simulink library "intertravamento"  (R2015a)
settings: Solver=ode45  SolverMode=SingleTasking  StartTime=0.0  StopTime=10.0  RelTol=1e-3
PostLoadFcn:
  | setsysloc_simulink(bdroot)
undefined symbols (not defined in the file or in its folder): docblock, getdatatypespecs, NumBits1, NumBits2, sfunxy, sigbuilder_block, slcm, SlDemoSign, Slope1, Slope2
libraries: simulink x46, sl_helperblocks x2, eml_lib x1
(part 2 of 6)

== system intertravamento/Continuous ==
  note: Integrators
  note: Delays
  note: Transfer Functions
  note: PID Controllers
  note: Derivative
  Derivative : Derivative
  Integrator : Integrator
  Integrator Limited : Integrator  LimitOutput=on  UpperSaturationLimit=1  LowerSaturationLimit=0
  "Integrator, Second-Order" : SecondOrderIntegrator
  "Integrator, Second-Order Limited" : SecondOrderIntegrator  LimitX=on  UpperLimitX=1  LowerLimitX=0  LimitDXDT=on
  PID Controller : Subsystem  DialogController=pidpack.PIDConfig.pidDDGCreate  mask(PID 1dof){Controller=PID, TimeDomain=Continuous-time, SampleTime=-1, IntegratorMethod=Forward Euler, FilterMethod=Forward Euler, Form=Parallel, UseFilter=on, ControllerParametersSource=internal, P=1, I=1, D=0, N=100, InitialConditionSource=internal, InitialConditionForIntegrator=0, InitialConditionForFilter=0, ExternalReset=none, IgnoreLimit=off, ZeroCross=on, LimitOutput=off, UpperSaturationLimit=inf, LowerSaturationLimit=-inf, LinearizeAsGain=on, AntiWindupMode=none, Kb=1, TrackingMode=off, Kt=1, RndMeth=Floor, SaturateOnIntegerOverflow=off, LockScale=off, PParamMin=[], PParamMax=[], PParamDataTypeStr=Inherit: Inherit via internal rule, IParamMin=[], IParamMax=[], IParamDataTypeStr=Inherit: Inherit via internal rule, DParamMin=[], DParamMax=[], DParamDataTypeStr=Inherit: Inherit via internal rule, NParamMin=[], NParamMax=[], NParamDataTypeStr=Inherit: Inherit via internal rule, KbParamMin=[], KbParamMax=[], KbParamDataTypeStr=Inherit: Inherit via internal rule, KtParamMin=[], KtParamMax=[], KtParamDataTypeStr=Inherit: Inherit via internal rule, POutMin=[], POutMax=[], POutDataTypeStr=Inherit: Inherit via internal rule, PGainOutDataTypeStr=Inherit: Inherit via internal rule, PProdOutDataTypeStr=Inherit: Inherit via internal rule, IOutMin=[], IOutMax=[], IOutDataTypeStr=Inherit: Inherit via internal rule, IGainOutDataTypeStr=Inherit: Inherit via internal rule, IProdOutDataTypeStr=Inherit: Inherit via internal rule, DOutMin=[], DOutMax=[], DOutDataTypeStr=Inherit: Inherit via internal rule, DGainOutDataTypeStr=Inherit: Inherit via internal rule, DProdOutDataTypeStr=Inherit: Inherit via internal rule, NOutMin=[], NOutMax=[], NOutDataTypeStr=Inherit: Inherit via internal rule, NGainOutDataTypeStr=Inherit: Inherit via internal rule, NProdOutDataTypeStr=Inherit: Inherit via internal rule, KbOutMin=[], KbOutMax=[], KbOutDataTypeStr=Inherit: Inherit via internal rule, KtOutMin=[], KtOutMax=[], KtOutDataTypeStr=Inherit: Inherit via internal rule, IntegratorOutMin=[], IntegratorOutMax=[], IntegratorOutDataTypeStr=Inherit: Inherit via internal rule, FilterOutMin=[], FilterOutMax=[], FilterOutDataTypeStr=Inherit: Inherit via internal rule, SumOutMin=[], SumOutMax=[], SumOutDataTypeStr=Inherit: Inherit via internal rule, SumI1OutMin=[], SumI1OutMax=[], SumI1OutDataTypeStr=Inherit: Inherit via internal rule, SumI2OutMin=[], SumI2OutMax=[], SumI2OutDataTypeStr=Inherit: Inherit via internal rule, SumI3OutMin=[], SumI3OutMax=[], SumI3OutDataTypeStr=Inherit: Inherit via internal rule, SumDOutMin=[], SumDOutMax=[], SumDOutDataTypeStr=Inherit: Inherit via internal rule, SumAccumDataTypeStr=Inherit: Inherit via internal rule, SumI1AccumDataTypeStr=Inherit: Inherit via internal rule, SumI2AccumDataTypeStr=Inherit: Inherit via internal rule, SumI3AccumDataTypeStr=Inherit: Inherit via internal rule, SumDAccumDataTypeStr=Inherit: Inherit via internal rule, SaturationOutMin=[], SaturationOutMax=[], SaturationOutDataTypeStr=Inherit: Same as input, IntegratorContinuousStateAttributes='', IntegratorStateIdentifier=, IntegratorStateMustResolveToSignalObject=off, IntegratorRTWStateStorageClass=Auto, IntegratorRTWStateStorageTypeQualifier=, FilterContinuousStateAttributes='', FilterStateIdentifier=, FilterStateMustResolveToSignalObject=off, FilterRTWStateStorageClass=Auto, FilterRTWStateStorageTypeQualifier=, DifferentiatorICPrevScaledInput=0, DifferentiatorOutMin=[], DifferentiatorOutMax=[], DifferentiatorOutDataTypeStr=Inherit: Inherit via internal rule}
      mask prompts: Controller "Simulink:masks:Controller_MP"; TimeDomain "Simulink:masks:TimeDomain_MP"; SampleTime "Simulink:masks:SampleTime1ForInherited_MP"; IntegratorMethod "Simulink:masks:IntegratorMethod_MP"; FilterMethod "Simulink:masks:FilterMethod_MP"; Form "Simulink:masks:Form_MP"; UseFilter "Simulink:masks:UseFilter_MP"; ControllerParametersSource "Simulink:masks:Source_MP"; P "Simulink:masks:ProportionalP_MP"; I "Simulink:masks:IntegralI_MP"; D "Simulink:masks:DerivativeD_MP"; N "Simulink:masks:FilterCoefficientN_MP"; InitialConditionSource "Simulink:masks:Source_MP"; InitialConditionForIntegrator "Simulink:masks:Integrator_MP"; InitialConditionForFilter "Simulink:masks:Filter_MP"; ExternalReset "Simulink:masks:ExternalReset_MP"; IgnoreLimit "Simulink:masks:IgnoreResetWhenLinearizing_MP"; ZeroCross "Simulink:masks:EnableZerocrossingDetection_MP"; LimitOutput "Simulink:masks:LimitOutput_MP"; UpperSaturationLimit "Simulink:masks:UpperSaturationLimit_MP"; LowerSaturationLimit "Simulink:masks:LowerSaturationLimit_MP"; LinearizeAsGain "Simulink:masks:IgnoreSaturationWhenLinearizing_MP"; AntiWindupMode "Simulink:masks:AntiwindupMethod_MP"; Kb "Simulink:masks:BackcalculationCoefficientKb_MP"; TrackingMode "Simulink:masks:EnableTrackingMode_MP"; Kt "Simulink:masks:TrackingCoefficientKt_MP"; RndMeth "Simulink:masks:IntegerRoundingMode_MP"; SaturateOnIntegerOverflow "Simulink:masks:SaturateOnIntegerOverflow_MP"; LockScale "Simulink:masks:LockDataTypeAgainstFxpTools_MP"; PParamMin "Simulink:masks:PParameterMinimum_MP"; PParamMax "Simulink:masks:PParameterMaximum_MP"; PParamDataTypeStr "Simulink:masks:PParameter_MP"; IParamMin "Simulink:masks:IParameterMinimum_MP"; IParamMax "Simulink:masks:IParameterMaximum_MP"; IParamDataTypeStr "Simulink:masks:IParameter_MP"; DParamMin "Simulink:masks:DParameterMinimum_MP"; DParamMax "Simulink:masks:DParameterMaximum_MP"; DParamDataTypeStr "Simulink:masks:DParameter_MP"; NParamMin "Simulink:masks:NParameterMinimum_MP"; NParamMax "Simulink:masks:NParameterMaximum_MP"; NParamDataTypeStr "Simulink:masks:NParameter_MP"; KbParamMin "Simulink:masks:KbParameterMinimum_MP"; KbParamMax "Simulink:masks:KbParameterMaximum_MP"; KbParamDataTypeStr "Simulink:masks:KbParameter_MP"; KtParamMin "Simulink:masks:KtParameterMinimum_MP"; KtParamMax "Simulink:masks:KtParameterMaximum_MP"; KtParamDataTypeStr "Simulink:masks:KtParameter_MP"; POutMin "Simulink:masks:PProductOutputMinimum_MP"; POutMax "Simulink:masks:PProductOutputMaximum_MP"; POutDataTypeStr "Simulink:masks:PProductOutput_MP"; PGainOutDataTypeStr "Simulink:masks:PProductOutput_MP"; PProdOutDataTypeStr "Simulink:masks:PProductOutput_MP"; IOutMin "Simulink:masks:IProductOutputMinimum_MP"; IOutMax "Simulink:masks:IProductOutputMaximum_MP"; IOutDataTypeStr "Simulink:masks:IProductOutput_MP"; IGainOutDataTypeStr "Simulink:masks:IProductOutput_MP"; IProdOutDataTypeStr "Simulink:masks:IProductOutput_MP"; DOutMin "Simulink:masks:DProductOutputMinimum_MP"; DOutMax "Simulink:masks:DProductOutputMaximum_MP"; DOutDataTypeStr "Simulink:masks:DProductOutput_MP"; DGainOutDataTypeStr "Simulink:masks:DProductOutput_MP"; DProdOutDataTypeStr "Simulink:masks:DProductOutput_MP"; NOutMin "Simulink:masks:NProductOutputMinimum_MP"; NOutMax "Simulink:masks:NProductOutputMaximum_MP"; NOutDataTypeStr "Simulink:masks:NProductOutput_MP"; NGainOutDataTypeStr "Simulink:masks:NProductOutput_MP"; NProdOutDataTypeStr "Simulink:masks:NProductOutput_MP"; KbOutMin "Simulink:masks:KbProductOutputMinimum_MP"; KbOutMax "Simulink:masks:KbProductOutputMaximum_MP"; KbOutDataTypeStr "Simulink:masks:KbProductOutput_MP"; KtOutMin "Simulink:masks:KtProductOutputMinimum_MP"; KtOutMax "Simulink:masks:KtProductOutputMaximum_MP"; KtOutDataTypeStr "Simulink:masks:KtProductOutput_MP"; IntegratorOutMin "Simulink:masks:IntegratorOutputMinimum_MP"; IntegratorOutMax "Simulink:masks:IntegratorOutputMaximum_MP"; IntegratorOutDataTypeStr "Simulink:masks:IntegratorOutput_MP"; FilterOutMin "Simulink:masks:FilterOutputMinimum_MP"; FilterOutMax "Simulink:masks:FilterOutputMaximum_MP"; FilterOutDataTypeStr "Simulink:masks:FilterOutput_MP"; SumOutMin "Simulink:masks:SumOutputMinimum_MP"; SumOutMax "Simulink:masks:SumOutputMaximum_MP"; SumOutDataTypeStr "Simulink:masks:SumOutput_MP"; SumI1OutMin "Simulink:masks:SumI1OutputMinimum_MP"; SumI1OutMax "Simulink:masks:SumI1OutputMaximum_MP"; SumI1OutDataTypeStr "Simulink:masks:SumI1Output_MP"; SumI2OutMin "Simulink:masks:SumI2OutputMinimum_MP"; SumI2OutMax "Simulink:masks:SumI2OutputMaximum_MP"; SumI2OutDataTypeStr "Simulink:masks:SumI2Output_MP"; SumI3OutMin "Simulink:masks:SumI3OutputMinimum_MP"; SumI3OutMax "Simulink:masks:SumI3OutputMaximum_MP"; SumI3OutDataTypeStr "Simulink:masks:SumI3Output_MP"; SumDOutMin "Simulink:masks:SumDOutputMinimum_MP"; SumDOutMax "Simulink:masks:SumDOutputMaximum_MP"; SumDOutDataTypeStr "Simulink:masks:SumDOutput_MP"; SumAccumDataTypeStr "Simulink:masks:AccumulatorOfSum_MP"; SumI1AccumDataTypeStr "Simulink:masks:AccumulatorOfSumI1_MP"; SumI2AccumDataTypeStr "Simulink:masks:AccumulatorOfSumI2_MP"; SumI3AccumDataTypeStr "Simulink:masks:AccumulatorOfSumI3_MP"; SumDAccumDataTypeStr "Simulink:masks:AccumulatorOfSumD_MP"; SaturationOutMin "Simulink:masks:SaturationOutputMinimum_MP"; SaturationOutMax "Simulink:masks:SaturationOutputMaximum_MP"; SaturationOutDataTypeStr "Simulink:masks:SaturationOutput_MP"; IntegratorContinuousStateAttributes "Simulink:masks:StateNameegposition_MP"; IntegratorStateIdentifier "Simulink:masks:StateName_MP"; IntegratorStateMustResolveToSignalObject "Simulink:masks:StateNameMustResolveToSimulinkSignalObject_MP"; IntegratorRTWStateStorageClass "Simulink:masks:CodeGenerationStorageClass_MP"; IntegratorRTWStateStorageTypeQualifier "Simulink:masks:CodeGenerationStorageTypeQualifier_MP"; FilterContinuousStateAttributes "Simulink:masks:StateNameegposition_MP"; FilterStateIdentifier "Simulink:masks:StateName_MP"; FilterStateMustResolveToSignalObject "Simulink:masks:StateNameMustResolveToSimulinkSignalObject_MP"; FilterRTWStateStorageClass "Simulink:masks:CodeGenerationStorageClass_MP"; FilterRTWStateStorageTypeQualifier "Simulink:masks:CodeGenerationStorageTypeQualifier_MP"; DifferentiatorICPrevScaledInput "Simulink:masks:Differentiator_MP"; DifferentiatorOutMin "Simulink:masks:DifferentiatorOutputMinimum_MP"; DifferentiatorOutMax "Simulink:masks:DifferentiatorOutputMaximum_MP"; DifferentiatorOutDataTypeStr "Simulink:masks:DifferentiatorOutput_MP"
      mask help: Simulink:masks:PID1dof_MD
      mask init:
      | pidpack.PIDConfig.configPID(gcbh);
      settings: DeleteFcn=pidpack.PIDConfig.closeTuner(gcbh)  ModelCloseFcn=pidpack.PIDConfig.closeTuner(gcbh)  NameChangeFcn=pidpack.PIDConfig.updateTunerName(gcbh)
      mask TypeOptions Controller: Simulink:masks:PID | Simulink:masks:PI | Simulink:masks:PD | Simulink:masks:P | Simulink:masks:I
      mask TypeOptions TimeDomain: Simulink:masks:ContinuousTime | Simulink:masks:DiscreteTime
      mask TypeOptions SampleTime: u/SampleTime | y/SampleTime | r/SampleTime | RESET/SampleTime | I0/SampleTime | D0/SampleTime | TR/SampleTime | Clamping circuit/preSat/SampleTime | Clamping circuit/preIntegrator/SampleTime | Clamping circuit/preP/SampleTime | Clamping circuit/AND/SampleTime | Clamping circuit/AND1/SampleTime | Clamping circuit/AND2/SampleTime | Clamping circuit/AND3/SampleTime | Clamping circuit/Gain/SampleTime | Clamping circuit/DataTypeConv2/SampleTime | Clamping circuit/DataTypeConv3/SampleTime | Clamping circuit/DeadZone/SampleTime | Clamping circuit/Equal/SampleTime | Clamping circuit/Equal1/SampleTime | Clamping circuit/Equal2/SampleTime | Clamping circuit/NOT1/SampleTime | Clamping circuit/NOT2/SampleTime | Clamping circuit/NotEqual/SampleTime | Clamping circuit/OR1/SampleTime | Clamping circuit/SignPreIntegrator/SampleTime | Clamping circuit/SignPreP/SampleTime | Clamping circuit/SignPreSat/SampleTime | Clamping circuit/Clamp/SampleTime | Derivative Gain/SampleTime | Filter/SampleTime | Filter Coefficient/SampleTime | Integral Gain/SampleTime | Integrator/SampleTime | Kb/SampleTime | Kt/SampleTime | Proportional Gain/SampleTime | Saturate/SampleTime | sprintf('/Setpoint Weighting\n(Derivative)')/SampleTime | sprintf('/Setpoint Weighting\n(Proportional)')/SampleTime | Sum/SampleTime | Sum1/SampleTime | Sum2/SampleTime | Sum3/SampleTime | SumD/SampleTime | SumI1/SampleTime | SumI2/SampleTime | SumI3/SampleTime | Switch/SampleTime | Differentiator/U/SampleTime | Differentiator/Y/SampleTime | POut/SampleTime | IOut/SampleTime | DOut/SampleTime | NOut/SampleTime | P/SampleTime | I/SampleTime | D/SampleTime | N/SampleTime
      mask TypeOptions IntegratorMethod: Simulink:masks:ForwardEuler | Simulink:masks:BackwardEuler | Simulink:masks:Trapezoidal
      mask TypeOptions FilterMethod: Simulink:masks:ForwardEuler | Simulink:masks:BackwardEuler | Simulink:masks:Trapezoidal
      mask TypeOptions Form: Simulink:masks:Ideal | Simulink:masks:Parallel
      mask TypeOptions ControllerParametersSource: Simulink:masks:internal | Simulink:masks:external
      mask TypeOptions P: Proportional Gain/Gain
      mask TypeOptions I: Integral Gain/Gain
      mask TypeOptions D: Derivative Gain/Gain
      mask TypeOptions N: Filter Coefficient/Gain
      mask TypeOptions InitialConditionSource: Simulink:masks:internal | Simulink:masks:external
      mask TypeOptions InitialConditionForIntegrator: Integrator/InitialCondition
      mask TypeOptions InitialConditionForFilter: Filter/InitialCondition
      mask TypeOptions ExternalReset: Simulink:masks:none | Simulink:masks:rising | Simulink:masks:falling | Simulink:masks:either | Simulink:masks:level
      mask TypeOptions UpperSaturationLimit: Clamping circuit/DeadZone/UpperValue | Saturate/UpperLimit
      mask TypeOptions LowerSaturationLimit: Clamping circuit/DeadZone/LowerValue | Saturate/LowerLimit
      mask TypeOptions AntiWindupMode: Simulink:masks:none | Simulink:masks:backCalculation | Simulink:masks:clamping
      mask TypeOptions Kb: Kb/Gain
      mask TypeOptions Kt: Kt/Gain
      mask TypeOptions RndMeth: Clamping circuit/Gain/RndMeth | Clamping circuit/DataTypeConv2/RndMeth | Clamping circuit/DataTypeConv3/RndMeth | Derivative Gain/RndMeth | Differentiator/RndMeth | Filter/RndMeth | Filter Coefficient/RndMeth | Integral Gain/RndMeth | Integrator/RndMeth | Kb/RndMeth | Kt/RndMeth | Proportional Gain/RndMeth | Saturate/RndMeth | sprintf('/Setpoint Weighting\n(Derivative)')/RndMeth | sprintf('/Setpoint Weighting\n(Proportional)')/RndMeth | Sum/RndMeth | Sum1/RndMeth | Sum2/RndMeth | Sum3/RndMeth | SumD/RndMeth | SumI1/RndMeth | SumI2/RndMeth | SumI3/RndMeth | Switch/RndMeth | Differentiator/TSamp/RndMeth | Differentiator/Diff/RndMeth | POut/RndMeth | IOut/RndMeth | DOut/RndMeth | NOut/RndMeth
      mask TypeOptions SaturateOnIntegerOverflow: Clamping circuit/Gain/SaturateOnIntegerOverflow | Clamping circuit/DataTypeConv2/SaturateOnIntegerOverflow | Clamping circuit/DataTypeConv3/SaturateOnIntegerOverflow | Clamping circuit/DeadZone/SaturateOnIntegerOverflow | Derivative Gain/SaturateOnIntegerOverflow | Filter/SaturateOnIntegerOverflow | Filter Coefficient/SaturateOnIntegerOverflow | Integral Gain/SaturateOnIntegerOverflow | Integrator/SaturateOnIntegerOverflow | Kb/SaturateOnIntegerOverflow | Kt/SaturateOnIntegerOverflow | Proportional Gain/SaturateOnIntegerOverflow | sprintf('/Setpoint Weighting\n(Derivative)')/SaturateOnIntegerOverflow | sprintf('/Setpoint Weighting\n(Proportional)')/SaturateOnIntegerOverflow | Sum/SaturateOnIntegerOverflow | Sum1/SaturateOnIntegerOverflow | Sum2/SaturateOnIntegerOverflow | Sum3/SaturateOnIntegerOverflow | SumD/SaturateOnIntegerOverflow | SumI1/SaturateOnIntegerOverflow | SumI2/SaturateOnIntegerOverflow | SumI3/SaturateOnIntegerOverflow | Switch/SaturateOnIntegerOverflow | Differentiator/TSamp/SaturateOnIntegerOverflow | Differentiator/Diff/SaturateOnIntegerOverflow | POut/SaturateOnIntegerOverflow | IOut/SaturateOnIntegerOverflow | DOut/SaturateOnIntegerOverflow | NOut/SaturateOnIntegerOverflow
      mask TypeOptions LockScale: Clamping circuit/preSat/LockScale | Clamping circuit/preIntegrator/LockScale | Clamping circuit/preP/LockScale | Clamping circuit/Gain/LockScale | Clamping circuit/DataTypeConv2/LockScale | Clamping circuit/DataTypeConv3/LockScale | Clamping circuit/Clamp/LockScale | Constant/LockScale | Derivative Gain/LockScale | Differentiator/LockScale | Filter/LockScale | Filter Coefficient/LockScale | Integral Gain/LockScale | Integrator/LockScale | Kb/LockScale | Kt/LockScale | Proportional Gain/LockScale | Saturate/LockScale | sprintf('/Setpoint Weighting\n(Derivative)')/LockScale | sprintf('/Setpoint Weighting\n(Proportional)')/LockScale | Sum/LockScale | Sum1/LockScale | Sum2/LockScale | Sum3/LockScale | SumD/LockScale | SumI1/LockScale | SumI2/LockScale | SumI3/LockScale | Switch/LockScale | Differentiator/U/LockScale | Differentiator/Diff/LockScale | Differentiator/Y/LockScale | POut/LockScale | IOut/LockScale | DOut/LockScale | NOut/LockScale
      mask TypeOptions PParamMin: Proportional Gain/ParamMin
      mask TypeOptions PParamMax: Proportional Gain/ParamMax
      mask TypeOptions PParamDataTypeStr: Proportional Gain/ParamDataTypeStr
      mask TypeOptions IParamMin: Integral Gain/ParamMin
      mask TypeOptions IParamMax: Integral Gain/ParamMax
      mask TypeOptions IParamDataTypeStr: Integral Gain/ParamDataTypeStr
      mask TypeOptions DParamMin: Derivative Gain/ParamMin
      mask TypeOptions DParamMax: Derivative Gain/ParamMax
      mask TypeOptions DParamDataTypeStr: Derivative Gain/ParamDataTypeStr
      mask TypeOptions NParamMin: Filter Coefficient/ParamMin
      mask TypeOptions NParamMax: Filter Coefficient/ParamMax
      mask TypeOptions NParamDataTypeStr: Filter Coefficient/ParamDataTypeStr
      mask TypeOptions KbParamMin: Kb/ParamMin
      mask TypeOptions KbParamMax: Kb/ParamMax
      mask TypeOptions KbParamDataTypeStr: Kb/ParamDataTypeStr
      mask TypeOptions KtParamMin: Kt/ParamMin
      mask TypeOptions KtParamMax: Kt/ParamMax
      mask TypeOptions KtParamDataTypeStr: Kt/ParamDataTypeStr
      mask TypeOptions POutMin: Proportional Gain/OutMin | POut/OutMin
      mask TypeOptions POutMax: Proportional Gain/OutMax | POut/OutMax
      mask TypeOptions PGainOutDataTypeStr: Proportional Gain/OutDataTypeStr
      mask TypeOptions PProdOutDataTypeStr: POut/OutDataTypeStr
      mask TypeOptions IOutMin: Integral Gain/OutMin | IOut/OutMin
      mask TypeOptions IOutMax: Integral Gain/OutMax | IOut/OutMax
      mask TypeOptions IGainOutDataTypeStr: Integral Gain/OutDataTypeStr
      mask TypeOptions IProdOutDataTypeStr: IOut/OutDataTypeStr
      mask TypeOptions DOutMin: Derivative Gain/OutMin | DOut/OutMin
      mask TypeOptions DOutMax: Derivative Gain/OutMax | DOut/OutMax
      mask TypeOptions DGainOutDataTypeStr: Derivative Gain/OutDataTypeStr
      mask TypeOptions DProdOutDataTypeStr: DOut/OutDataTypeStr
      mask TypeOptions NOutMin: Filter Coefficient/OutMin | NOut/OutMin
      mask TypeOptions NOutMax: Filter Coefficient/OutMax | NOut/OutMax
      mask TypeOptions NGainOutDataTypeStr: Filter Coefficient/OutDataTypeStr
      mask TypeOptions NProdOutDataTypeStr: NOut/OutDataTypeStr
      mask TypeOptions KbOutMin: Kb/OutMin
      mask TypeOptions KbOutMax: Kb/OutMax
      mask TypeOptions KbOutDataTypeStr: Kb/OutDataTypeStr
      mask TypeOptions KtOutMin: Kt/OutMin
      mask TypeOptions KtOutMax: Kt/OutMax
      mask TypeOptions KtOutDataTypeStr: Kt/OutDataTypeStr
      mask TypeOptions IntegratorOutMin: Integrator/OutMin
      mask TypeOptions IntegratorOutMax: Integrator/OutMax
      mask TypeOptions IntegratorOutDataTypeStr: Integrator/OutDataTypeStr
      mask TypeOptions FilterOutMin: Filter/OutMin
      mask TypeOptions FilterOutMax: Filter/OutMax
      mask TypeOptions FilterOutDataTypeStr: Filter/OutDataTypeStr
      mask TypeOptions SumOutMin: Sum/OutMin
      mask TypeOptions SumOutMax: Sum/OutMax
      mask TypeOptions SumOutDataTypeStr: Sum/OutDataTypeStr
      mask TypeOptions SumI1OutMin: SumI1/OutMin
      mask TypeOptions SumI1OutMax: SumI1/OutMax
      mask TypeOptions SumI1OutDataTypeStr: SumI1/OutDataTypeStr
      mask TypeOptions SumI2OutMin: SumI2/OutMin
      mask TypeOptions SumI2OutMax: SumI2/OutMax
      mask TypeOptions SumI2OutDataTypeStr: SumI2/OutDataTypeStr
      mask TypeOptions SumI3OutMin: SumI3/OutMin
      mask TypeOptions SumI3OutMax: SumI3/OutMax
      mask TypeOptions SumI3OutDataTypeStr: SumI3/OutDataTypeStr
      mask TypeOptions SumDOutMin: SumD/OutMin
      mask TypeOptions SumDOutMax: SumD/OutMax
      mask TypeOptions SumDOutDataTypeStr: SumD/OutDataTypeStr
      mask TypeOptions SumAccumDataTypeStr: Sum/AccumDataTypeStr
      mask TypeOptions SumI1AccumDataTypeStr: SumI1/AccumDataTypeStr
      mask TypeOptions SumI2AccumDataTypeStr: SumI2/AccumDataTypeStr
      mask TypeOptions SumI3AccumDataTypeStr: SumI3/AccumDataTypeStr
      mask TypeOptions SumDAccumDataTypeStr: SumD/AccumDataTypeStr
      mask TypeOptions SaturationOutMin: Saturate/OutMin
      mask TypeOptions SaturationOutMax: Saturate/OutMax
      mask TypeOptions SaturationOutDataTypeStr: Saturate/OutDataTypeStr
      mask TypeOptions IntegratorContinuousStateAttributes: Integrator/ContinuousStateAttributes
      mask TypeOptions IntegratorStateIdentifier: Integrator/StateIdentifier
      mask TypeOptions IntegratorRTWStateStorageClass: Simulink:masks:Auto | Simulink:masks:ExportedGlobal | Simulink:masks:ImportedExtern | Simulink:masks:ImportedExternPointer
      mask TypeOptions FilterContinuousStateAttributes: Filter/ContinuousStateAttributes
      mask TypeOptions FilterStateIdentifier: Filter/StateIdentifier
      mask TypeOptions FilterRTWStateStorageClass: Simulink:masks:Auto | Simulink:masks:ExportedGlobal | Simulink:masks:ImportedExtern | Simulink:masks:ImportedExternPointer
      mask TypeOptions DifferentiatorICPrevScaledInput: Differentiator/UD/InitialCondition
      mask Display:
      | image(imread(fullfile(matlabroot,'toolbox','simulink','blocks','@pidpack','@PIDMasks','images','blank.png'),'png'),[0 0 1 1]);
      | disp('PID(s)')
      | port_label('input', 1, '');
      | port_label('output', 1, '');
  PID Controller (2DOF) : Subsystem  DialogController=pidpack.PIDConfig.pidDDGCreate  mask(PID 2dof){Controller=PID, TimeDomain=Continuous-time, SampleTime=-1, IntegratorMethod=Forward Euler, FilterMethod=Forward Euler, Form=Parallel, UseFilter=on, ControllerParametersSource=internal, P=1, I=1, D=0, N=100, b=1, c=1, InitialConditionSource=internal, InitialConditionForIntegrator=0, InitialConditionForFilter=0, ExternalReset=none, IgnoreLimit=off, ZeroCross=on, LimitOutput=off, UpperSaturationLimit=inf, LowerSaturationLimit=-inf, LinearizeAsGain=on, AntiWindupMode=none, Kb=1, TrackingMode=off, Kt=1, RndMeth=Floor, SaturateOnIntegerOverflow=off, LockScale=off, PParamMin=[], PParamMax=[], PParamDataTypeStr=Inherit: Inherit via internal rule, IParamMin=[], IParamMax=[], IParamDataTypeStr=Inherit: Inherit via internal rule, DParamMin=[], DParamMax=[], DParamDataTypeStr=Inherit: Inherit via internal rule, NParamMin=[], NParamMax=[], NParamDataTypeStr=Inherit: Inherit via internal rule, bParamMin=[], bParamMax=[], bParamDataTypeStr=Inherit: Inherit via internal rule, cParamMin=[], cParamMax=[], cParamDataTypeStr=Inherit: Inherit via internal rule, KbParamMin=[], KbParamMax=[], KbParamDataTypeStr=Inherit: Inherit via internal rule, KtParamMin=[], KtParamMax=[], KtParamDataTypeStr=Inherit: Inherit via internal rule, POutMin=[], POutMax=[], POutDataTypeStr=Inherit: Inherit via internal rule, PGainOutDataTypeStr=Inherit: Inherit via internal rule, PProdOutDataTypeStr=Inherit: Inherit via internal rule, IOutMin=[], IOutMax=[], IOutDataTypeStr=Inherit: Inherit via internal rule, IGainOutDataTypeStr=Inherit: Inherit via internal rule, IProdOutDataTypeStr=Inherit: Inherit via internal rule, DOutMin=[], DOutMax=[], DOutDataTypeStr=Inherit: Inherit via internal rule, DGainOutDataTypeStr=Inherit: Inherit via internal rule, DProdOutDataTypeStr=Inherit: Inherit via internal rule, NOutMin=[], NOutMax=[], NOutDataTypeStr=Inherit: Inherit via internal rule, NGainOutDataTypeStr=Inherit: Inherit via internal rule, NProdOutDataTypeStr=Inherit: Inherit via internal rule, bOutMin=[], bOutMax=[], bOutDataTypeStr=Inherit: Inherit via internal rule, bGainOutDataTypeStr=Inherit: Inherit via internal rule, bProdOutDataTypeStr=Inherit: Inherit via internal rule, cOutMin=[], cOutMax=[], cOutDataTypeStr=Inherit: Inherit via internal rule, cGainOutDataTypeStr=Inherit: Inherit via internal rule, cProdOutDataTypeStr=Inherit: Inherit via internal rule, KbOutMin=[], KbOutMax=[], KbOutDataTypeStr=Inherit: Inherit via internal rule, KtOutMin=[], KtOutMax=[], KtOutDataTypeStr=Inherit: Inherit via internal rule, IntegratorOutMin=[], IntegratorOutMax=[], IntegratorOutDataTypeStr=Inherit: Inherit via internal rule, FilterOutMin=[], FilterOutMax=[], FilterOutDataTypeStr=Inherit: Inherit via internal rule, SumOutMin=[], SumOutMax=[], SumOutDataTypeStr=Inherit: Inherit via internal rule, Sum1OutMin=[], Sum1OutMax=[], Sum1OutDataTypeStr=Inherit: Inherit via internal rule, Sum2OutMin=[], Sum2OutMax=[], Sum2OutDataTypeStr=Inherit: Inherit via internal rule, Sum3OutMin=[], Sum3OutMax=[], Sum3OutDataTypeStr=Inherit: Inherit via internal rule, SumI1OutMin=[], SumI1OutMax=[], SumI1OutDataTypeStr=Inherit: Inherit via internal rule, SumI2OutMin=[], SumI2OutMax=[], SumI2OutDataTypeStr=Inherit: Inherit via internal rule, SumI3OutMin=[], SumI3OutMax=[], SumI3OutDataTypeStr=Inherit: Inherit via internal rule, SumDOutMin=[], SumDOutMax=[], SumDOutDataTypeStr=Inherit: Inherit via internal rule, SumAccumDataTypeStr=Inherit: Inherit via internal rule, Sum1AccumDataTypeStr=Inherit: Inherit via internal rule, Sum2AccumDataTypeStr=Inherit: Inherit via internal rule, Sum3AccumDataTypeStr=Inherit: Inherit via internal rule, SumI1AccumDataTypeStr=Inherit: Inherit via internal rule, SumI2AccumDataTypeStr=Inherit: Inherit via internal rule, SumI3AccumDataTypeStr=Inherit: Inherit via internal rule, SumDAccumDataTypeStr=Inherit: Inherit via internal rule, SaturationOutMin=[], SaturationOutMax=[], SaturationOutDataTypeStr=Inherit: Same as input, IntegratorContinuousStateAttributes='', IntegratorStateIdentifier=, IntegratorStateMustResolveToSignalObject=off, IntegratorRTWStateStorageClass=Auto, IntegratorRTWStateStorageTypeQualifier=, FilterContinuousStateAttributes='', FilterStateIdentifier=, FilterStateMustResolveToSignalObject=off, FilterRTWStateStorageClass=Auto, FilterRTWStateStorageTypeQualifier=, DifferentiatorICPrevScaledInput=0, DifferentiatorOutMin=[], DifferentiatorOutMax=[], DifferentiatorOutDataTypeStr=Inherit: Inherit via internal rule}
      mask prompts: Controller "Simulink:masks:Controller_MP"; TimeDomain "Simulink:masks:TimeDomain_MP"; SampleTime "Simulink:masks:SampleTime1ForInherited_MP"; IntegratorMethod "Simulink:masks:IntegratorMethod_MP"; FilterMethod "Simulink:masks:FilterMethod_MP"; Form "Simulink:masks:Form_MP"; UseFilter "Simulink:masks:UseFilter_MP"; ControllerParametersSource "Simulink:masks:Source_MP"; P "Simulink:masks:ProportionalP_MP"; I "Simulink:masks:IntegralI_MP"; D "Simulink:masks:DerivativeD_MP"; N "Simulink:masks:FilterCoefficientN_MP"; b "Simulink:masks:SetpointWeightb_MP"; c "Simulink:masks:SetpointWeightc_MP"; InitialConditionSource "Simulink:masks:Source_MP"; InitialConditionForIntegrator "Simulink:masks:Integrator_MP"; InitialConditionForFilter "Simulink:masks:Filter_MP"; ExternalReset "Simulink:masks:ExternalReset_MP"; IgnoreLimit "Simulink:masks:IgnoreResetWhenLinearizing_MP"; ZeroCross "Simulink:masks:EnableZerocrossingDetection_MP"; LimitOutput "Simulink:masks:LimitOutput_MP"; UpperSaturationLimit "Simulink:masks:UpperSaturationLimit_MP"; LowerSaturationLimit "Simulink:masks:LowerSaturationLimit_MP"; LinearizeAsGain "Simulink:masks:IgnoreSaturationWhenLinearizing_MP"; AntiWindupMode "Simulink:masks:AntiwindupMethod_MP"; Kb "Simulink:masks:BackcalculationCoefficientKb_MP"; TrackingMode "Simulink:masks:EnableTrackingMode_MP"; Kt "Simulink:masks:TrackingCoefficientKt_MP"; RndMeth "Simulink:masks:IntegerRoundingMode_MP"; SaturateOnIntegerOverflow "Simulink:masks:SaturateOnIntegerOverflow_MP"; LockScale "Simulink:masks:LockDataTypeAgainstFxpTools_MP"; PParamMin "Simulink:masks:PParameterMinimum_MP"; PParamMax "Simulink:masks:PParameterMaximum_MP"; PParamDataTypeStr "Simulink:masks:PParameter_MP"; IParamMin "Simulink:masks:IParameterMinimum_MP"; IParamMax "Simulink:masks:IParameterMaximum_MP"; IParamDataTypeStr "Simulink:masks:IParameter_MP"; DParamMin "Simulink:masks:DParameterMinimum_MP"; DParamMax "Simulink:masks:DParameterMaximum_MP"; DParamDataTypeStr "Simulink:masks:DParameter_MP"; NParamMin "Simulink:masks:NParameterMinimum_MP"; NParamMax "Simulink:masks:NParameterMaximum_MP"; NParamDataTypeStr "Simulink:masks:NParameter_MP"; bParamMin "Simulink:masks:bParameterMinimum_MP"; bParamMax "Simulink:masks:bParameterMaximum_MP"; bParamDataTypeStr "Simulink:masks:bParameter_MP"; cParamMin "Simulink:masks:cParameterMinimum_MP"; cParamMax "Simulink:masks:cParameterMaximum_MP"; cParamDataTypeStr "Simulink:masks:cParameter_MP"; KbParamMin "Simulink:masks:KbParameterMinimum_MP"; KbParamMax "Simulink:masks:KbParameterMaximum_MP"; KbParamDataTypeStr "Simulink:masks:KbParameter_MP"; KtParamMin "Simulink:masks:KtParameterMinimum_MP"; KtParamMax "Simulink:masks:KtParameterMaximum_MP"; KtParamDataTypeStr "Simulink:masks:KtParameter_MP"; POutMin "Simulink:masks:PProductOutputMinimum_MP"; POutMax "Simulink:masks:PProductOutputMaximum_MP"; POutDataTypeStr "Simulink:masks:PProductOutput_MP"; PGainOutDataTypeStr "Simulink:masks:PProductOutput_MP"; PProdOutDataTypeStr "Simulink:masks:PProductOutput_MP"; IOutMin "Simulink:masks:IProductOutputMinimum_MP"; IOutMax "Simulink:masks:IProductOutputMaximum_MP"; IOutDataTypeStr "Simulink:masks:IProductOutput_MP"; IGainOutDataTypeStr "Simulink:masks:IProductOutput_MP"; IProdOutDataTypeStr "Simulink:masks:IProductOutput_MP"; DOutMin "Simulink:masks:DProductOutputMinimum_MP"; DOutMax "Simulink:masks:DProductOutputMaximum_MP"; DOutDataTypeStr "Simulink:masks:DProductOutput_MP"; DGainOutDataTypeStr "Simulink:masks:DProductOutput_MP"; DProdOutDataTypeStr "Simulink:masks:DProductOutput_MP"; NOutMin "Simulink:masks:NProductOutputMinimum_MP"; NOutMax "Simulink:masks:NProductOutputMaximum_MP"; NOutDataTypeStr "Simulink:masks:NProductOutput_MP"; NGainOutDataTypeStr "Simulink:masks:NProductOutput_MP"; NProdOutDataTypeStr "Simulink:masks:NProductOutput_MP"; bOutMin "Simulink:masks:bProductOutputMinimum_MP"; bOutMax "Simulink:masks:bProductOutputMaximum_MP"; bOutDataTypeStr "Simulink:masks:bProductOutput_MP"; bGainOutDataTypeStr "Simulink:masks:bProductOutput_MP"; bProdOutDataTypeStr "Simulink:masks:bProductOutput_MP"; cOutMin "Simulink:masks:cProductOutputMinimum_MP"; cOutMax "Simulink:masks:cProductOutputMaximum_MP"; cOutDataTypeStr "Simulink:masks:cProductOutput_MP"; cGainOutDataTypeStr "Simulink:masks:cProductOutput_MP"; cProdOutDataTypeStr "Simulink:masks:cProductOutput_MP"; KbOutMin "Simulink:masks:KbProductOutputMinimum_MP"; KbOutMax "Simulink:masks:KbProductOutputMaximum_MP"; KbOutDataTypeStr "Simulink:masks:KbProductOutput_MP"; KtOutMin "Simulink:masks:KtProductOutputMinimum_MP"; KtOutMax "Simulink:masks:KtProductOutputMaximum_MP"; KtOutDataTypeStr "Simulink:masks:KtProductOutput_MP"; IntegratorOutMin "Simulink:masks:IntegratorOutputMinimum_MP"; IntegratorOutMax "Simulink:masks:IntegratorOutputMaximum_MP"; IntegratorOutDataTypeStr "Simulink:masks:IntegratorOutput_MP"; FilterOutMin "Simulink:masks:FilterOutputMinimum_MP"; FilterOutMax "Simulink:masks:FilterOutputMaximum_MP"; FilterOutDataTypeStr "Simulink:masks:FilterOutput_MP"; SumOutMin "Simulink:masks:SumOutputMinimum_MP"; SumOutMax "Simulink:masks:SumOutputMaximum_MP"; SumOutDataTypeStr "Simulink:masks:SumOutput_MP"; Sum1OutMin "Simulink:masks:Sum1OutputMinimum_MP"; Sum1OutMax "Simulink:masks:Sum1OutputMaximum_MP"; Sum1OutDataTypeStr "Simulink:masks:Sum1Output_MP"; Sum2OutMin "Simulink:masks:Sum2OutputMinimum_MP"; Sum2OutMax "Simulink:masks:Sum2OutputMaximum_MP"; Sum2OutDataTypeStr "Simulink:masks:Sum2Output_MP"; Sum3OutMin "Simulink:masks:Sum3OutputMinimum_MP"; Sum3OutMax "Simulink:masks:Sum3OutputMaximum_MP"; Sum3OutDataTypeStr "Simulink:masks:Sum3Output_MP"; SumI1OutMin "Simulink:masks:SumI1OutputMinimum_MP"; SumI1OutMax "Simulink:masks:SumI1OutputMaximum_MP"; SumI1OutDataTypeStr "Simulink:masks:SumI1Output_MP"; SumI2OutMin "Simulink:masks:SumI2OutputMinimum_MP"; SumI2OutMax "Simulink:masks:SumI2OutputMaximum_MP"; SumI2OutDataTypeStr "Simulink:masks:SumI2Output_MP"; SumI3OutMin "Simulink:masks:SumI3OutputMinimum_MP"; SumI3OutMax "Simulink:masks:SumI3OutputMaximum_MP"; SumI3OutDataTypeStr "Simulink:masks:SumI3Output_MP"; SumDOutMin "Simulink:masks:SumDOutputMinimum_MP"; SumDOutMax "Simulink:masks:SumDOutputMaximum_MP"; SumDOutDataTypeStr "Simulink:masks:SumDOutput_MP"; SumAccumDataTypeStr "Simulink:masks:AccumulatorOfSum_MP"; Sum1AccumDataTypeStr "Simulink:masks:AccumulatorOfSum1_MP"; Sum2AccumDataTypeStr "Simulink:masks:AccumulatorOfSum2_MP"; Sum3AccumDataTypeStr "Simulink:masks:AccumulatorOfSum3_MP"; SumI1AccumDataTypeStr "Simulink:masks:AccumulatorOfSumI1_MP"; SumI2AccumDataTypeStr "Simulink:masks:AccumulatorOfSumI2_MP"; SumI3AccumDataTypeStr "Simulink:masks:AccumulatorOfSumI3_MP"; SumDAccumDataTypeStr "Simulink:masks:AccumulatorOfSumD_MP"; SaturationOutMin "Simulink:masks:SaturationOutputMinimum_MP"; SaturationOutMax "Simulink:masks:SaturationOutputMaximum_MP"; SaturationOutDataTypeStr "Simulink:masks:SaturationOutput_MP"; IntegratorContinuousStateAttributes "Simulink:masks:StateNameegposition_MP"; IntegratorStateIdentifier "Simulink:masks:StateName_MP"; IntegratorStateMustResolveToSignalObject "Simulink:masks:StateNameMustResolveToSimulinkSignalObject_MP"; IntegratorRTWStateStorageClass "Simulink:masks:CodeGenerationStorageClass_MP"; IntegratorRTWStateStorageTypeQualifier "Simulink:masks:CodeGenerationStorageTypeQualifier_MP"; FilterContinuousStateAttributes "Simulink:masks:StateNameegposition_MP"; FilterStateIdentifier "Simulink:masks:StateName_MP"; FilterStateMustResolveToSignalObject "Simulink:masks:StateNameMustResolveToSimulinkSignalObject_MP"; FilterRTWStateStorageClass "Simulink:masks:CodeGenerationStorageClass_MP"; FilterRTWStateStorageTypeQualifier "Simulink:masks:CodeGenerationStorageTypeQualifier_MP"; DifferentiatorICPrevScaledInput "Simulink:masks:Differentiator_MP"; DifferentiatorOutMin "Simulink:masks:DifferentiatorOutputMinimum_MP"; DifferentiatorOutMax "Simulink:masks:DifferentiatorOutputMaximum_MP"; DifferentiatorOutDataTypeStr "Simulink:masks:DifferentiatorOutput_MP"
      mask help: Simulink:masks:PID2dof_MD
      mask init:
      | pidpack.PIDConfig.configPID2DOF(gcbh);
      settings: DeleteFcn=pidpack.PIDConfig.closeTuner(gcbh)  ModelCloseFcn=pidpack.PIDConfig.closeTuner(gcbh)  NameChangeFcn=pidpack.PIDConfig.updateTunerName(gcbh)
      mask TypeOptions Controller: Simulink:masks:PID | Simulink:masks:PI | Simulink:masks:PD
      mask TypeOptions TimeDomain: Simulink:masks:ContinuousTime | Simulink:masks:DiscreteTime
      mask TypeOptions SampleTime: u/SampleTime | y/SampleTime | r/SampleTime | RESET/SampleTime | I0/SampleTime | D0/SampleTime | TR/SampleTime | Clamping circuit/preSat/SampleTime | Clamping circuit/preIntegrator/SampleTime | Clamping circuit/preP/SampleTime | Clamping circuit/AND/SampleTime | Clamping circuit/AND1/SampleTime | Clamping circuit/AND2/SampleTime | Clamping circuit/AND3/SampleTime | Clamping circuit/Gain/SampleTime | Clamping circuit/DataTypeConv2/SampleTime | Clamping circuit/DataTypeConv3/SampleTime | Clamping circuit/DeadZone/SampleTime | Clamping circuit/Equal/SampleTime | Clamping circuit/Equal1/SampleTime | Clamping circuit/Equal2/SampleTime | Clamping circuit/NOT1/SampleTime | Clamping circuit/NOT2/SampleTime | Clamping circuit/NotEqual/SampleTime | Clamping circuit/OR1/SampleTime | Clamping circuit/SignPreIntegrator/SampleTime | Clamping circuit/SignPreP/SampleTime | Clamping circuit/SignPreSat/SampleTime | Clamping circuit/Clamp/SampleTime | Derivative Gain/SampleTime | Filter/SampleTime | Filter Coefficient/SampleTime | Integral Gain/SampleTime | Integrator/SampleTime | Kb/SampleTime | Kt/SampleTime | Proportional Gain/SampleTime | Saturate/SampleTime | Setpoint Weighting (Derivative)/SampleTime | Setpoint Weighting (Proportional)/SampleTime | Sum/SampleTime | Sum1/SampleTime | Sum2/SampleTime | Sum3/SampleTime | SumD/SampleTime | SumI1/SampleTime | SumI2/SampleTime | SumI3/SampleTime | Switch/SampleTime | Differentiator/U/SampleTime | Differentiator/Y/SampleTime | POut/SampleTime | IOut/SampleTime | DOut/SampleTime | NOut/SampleTime | bOut/SampleTime | cOut/SampleTime | P/SampleTime | I/SampleTime | D/SampleTime | N/SampleTime | b/SampleTime | c/SampleTime
      mask TypeOptions IntegratorMethod: Simulink:masks:ForwardEuler | Simulink:masks:BackwardEuler | Simulink:masks:Trapezoidal
      mask TypeOptions FilterMethod: Simulink:masks:ForwardEuler | Simulink:masks:BackwardEuler | Simulink:masks:Trapezoidal
      mask TypeOptions Form: Simulink:masks:Ideal | Simulink:masks:Parallel
      mask TypeOptions ControllerParametersSource: Simulink:masks:internal | Simulink:masks:external
      mask TypeOptions P: Proportional Gain/Gain
      mask TypeOptions I: Integral Gain/Gain
      mask TypeOptions D: Derivative Gain/Gain
      mask TypeOptions N: Filter Coefficient/Gain
      mask TypeOptions b: Setpoint Weighting (Proportional)/Gain
      mask TypeOptions c: Setpoint Weighting (Derivative)/Gain
      mask TypeOptions InitialConditionSource: Filter/InitialConditionSource | Integrator/InitialConditionSource
      mask TypeOptions InitialConditionForIntegrator: Integrator/InitialCondition
      mask TypeOptions InitialConditionForFilter: Filter/InitialCondition
      mask TypeOptions ExternalReset: Simulink:masks:none | Simulink:masks:rising | Simulink:masks:falling | Simulink:masks:either | Simulink:masks:level
      mask TypeOptions UpperSaturationLimit: Clamping circuit/DeadZone/UpperValue | Saturate/UpperLimit
      mask TypeOptions LowerSaturationLimit: Clamping circuit/DeadZone/LowerValue | Saturate/LowerLimit
      mask TypeOptions AntiWindupMode: Simulink:masks:none | Simulink:masks:backCalculation | Simulink:masks:clamping
      mask TypeOptions Kb: Kb/Gain
      mask TypeOptions Kt: Kt/Gain
      mask TypeOptions RndMeth: Clamping circuit/Gain/RndMeth | Clamping circuit/DataTypeConv2/RndMeth | Clamping circuit/DataTypeConv3/RndMeth | Derivative Gain/RndMeth | Differentiator/RndMeth | Filter/RndMeth | Filter Coefficient/RndMeth | Integral Gain/RndMeth | Integrator/RndMeth | Kb/RndMeth | Kt/RndMeth | Proportional Gain/RndMeth | Saturate/RndMeth | Setpoint Weighting (Derivative)/RndMeth | Setpoint Weighting (Proportional)/RndMeth | Sum/RndMeth | Sum1/RndMeth | Sum2/RndMeth | Sum3/RndMeth | SumD/RndMeth | SumI1/RndMeth | SumI2/RndMeth | SumI3/RndMeth | Switch/RndMeth | Differentiator/U/LockScale | Differentiator/Diff/RndMeth | POut/RndMeth | IOut/RndMeth | DOut/RndMeth | NOut/RndMeth | bOut/RndMeth | cOut/RndMeth
      mask TypeOptions SaturateOnIntegerOverflow: Clamping circuit/Gain/SaturateOnIntegerOverflow | Clamping circuit/DataTypeConv2/SaturateOnIntegerOverflow | Clamping circuit/DataTypeConv3/SaturateOnIntegerOverflow | Clamping circuit/DeadZone/SaturateOnIntegerOverflow | Derivative Gain/SaturateOnIntegerOverflow | Filter/SaturateOnIntegerOverflow | Filter Coefficient/SaturateOnIntegerOverflow | Integral Gain/SaturateOnIntegerOverflow | Integrator/SaturateOnIntegerOverflow | Kb/SaturateOnIntegerOverflow | Kt/SaturateOnIntegerOverflow | Proportional Gain/SaturateOnIntegerOverflow | Setpoint Weighting (Derivative)/SaturateOnIntegerOverflow | Setpoint Weighting (Proportional)/SaturateOnIntegerOverflow | Sum/SaturateOnIntegerOverflow | Sum1/SaturateOnIntegerOverflow | Sum2/SaturateOnIntegerOverflow | Sum3/SaturateOnIntegerOverflow | SumD/SaturateOnIntegerOverflow | SumI1/SaturateOnIntegerOverflow | SumI2/SaturateOnIntegerOverflow | SumI3/SaturateOnIntegerOverflow | Switch/SaturateOnIntegerOverflow | Differentiator/Diff/SaturateOnIntegerOverflow | POut/SaturateOnIntegerOverflow | IOut/SaturateOnIntegerOverflow | DOut/SaturateOnIntegerOverflow | NOut/SaturateOnIntegerOverflow | bOut/SaturateOnIntegerOverflow | cOut/SaturateOnIntegerOverflow
      mask TypeOptions LockScale: Clamping circuit/preSat/LockScale | Clamping circuit/preIntegrator/LockScale | Clamping circuit/preP/LockScale | Clamping circuit/Gain/LockScale | Clamping circuit/DataTypeConv2/LockScale | Clamping circuit/DataTypeConv3/LockScale | Clamping circuit/Clamp/LockScale | Constant/LockScale | Derivative Gain/LockScale | Differentiator/LockScale | Filter/LockScale | Filter Coefficient/LockScale | Integral Gain/LockScale | Integrator/LockScale | Kb/LockScale | Kt/LockScale | Proportional Gain/LockScale | Saturate/LockScale | Setpoint Weighting (Derivative)/LockScale | Setpoint Weighting (Proportional)/LockScale | Sum/LockScale | Sum1/LockScale | Sum2/LockScale | Sum3/LockScale | SumD/LockScale | SumI1/LockScale | SumI2/LockScale | SumI3/LockScale | Switch/LockScale | Differentiator/Diff/LockScale | Differentiator/Y/LockScale | POut/LockScale | IOut/LockScale | DOut/LockScale | NOut/LockScale | bOut/LockScale | cOut/LockScale
      mask TypeOptions PParamMin: Proportional Gain/ParamMin
      mask TypeOptions PParamMax: Proportional Gain/ParamMax
      mask TypeOptions PParamDataTypeStr: Proportional Gain/ParamDataTypeStr
      mask TypeOptions IParamMin: Integral Gain/ParamMin
      mask TypeOptions IParamMax: Integral Gain/ParamMax
      mask TypeOptions IParamDataTypeStr: Integral Gain/ParamDataTypeStr
      mask TypeOptions DParamMin: Derivative Gain/ParamMin
      mask TypeOptions DParamMax: Derivative Gain/ParamMax
      mask TypeOptions DParamDataTypeStr: Derivative Gain/ParamDataTypeStr
      mask TypeOptions NParamMin: Filter Coefficient/ParamMin
      mask TypeOptions NParamMax: Filter Coefficient/ParamMax
      mask TypeOptions NParamDataTypeStr: Filter Coefficient/ParamDataTypeStr
      mask TypeOptions bParamMin: Setpoint Weighting (Proportional)/ParamMin
      mask TypeOptions bParamMax: Setpoint Weighting (Proportional)/ParamMax
      mask TypeOptions bParamDataTypeStr: Setpoint Weighting (Proportional)/ParamDataTypeStr
      mask TypeOptions cParamMin: Setpoint Weighting (Derivative)/ParamMin
      mask TypeOptions cParamMax: Setpoint Weighting (Derivative)/ParamMax
      mask TypeOptions cParamDataTypeStr: Setpoint Weighting (Derivative)/ParamDataTypeStr
      mask TypeOptions KbParamMin: Kb/ParamMin
      mask TypeOptions KbParamMax: Kb/ParamMax
      mask TypeOptions KbParamDataTypeStr: Kb/ParamDataTypeStr
      mask TypeOptions KtParamMin: Kt/ParamMin
      mask TypeOptions KtParamMax: Kt/ParamMax
      mask TypeOptions KtParamDataTypeStr: Kt/ParamDataTypeStr
      mask TypeOptions POutMin: Proportional Gain/OutMin | POut/OutMin
      mask TypeOptions POutMax: Proportional Gain/OutMax | POut/OutMax
      mask TypeOptions PGainOutDataTypeStr: Proportional Gain/OutDataTypeStr
      mask TypeOptions PProdOutDataTypeStr: POut/OutDataTypeStr
      mask TypeOptions IOutMin: Integral Gain/OutMin | IOut/OutMin
      mask TypeOptions IOutMax: Integral Gain/OutMax | IOut/OutMax
      mask TypeOptions IGainOutDataTypeStr: Integral Gain/OutDataTypeStr
      mask TypeOptions IProdOutDataTypeStr: IOut/OutDataTypeStr
      mask TypeOptions DOutMin: Derivative Gain/OutMin | DOut/OutMin
      mask TypeOptions DOutMax: Derivative Gain/OutMax | DOut/OutMax
      mask TypeOptions DGainOutDataTypeStr: Derivative Gain/OutDataTypeStr
      mask TypeOptions DProdOutDataTypeStr: DOut/OutDataTypeStr
      mask TypeOptions NOutMin: Filter Coefficient/OutMin | NOut/OutMin
      mask TypeOptions NOutMax: Filter Coefficient/OutMax | NOut/OutMax
      mask TypeOptions NGainOutDataTypeStr: Filter Coefficient/OutDataTypeStr
      mask TypeOptions NProdOutDataTypeStr: NOut/OutDataTypeStr
      mask TypeOptions bOutMin: Setpoint Weighting (Proportional)/OutMin | bOut/OutMin
      mask TypeOptions bOutMax: Setpoint Weighting (Proportional)/OutMax | bOut/OutMax
      mask TypeOptions bGainOutDataTypeStr: Setpoint Weighting (Proportional)/OutDataTypeStr
      mask TypeOptions bProdOutDataTypeStr: bOut/OutDataTypeStr
      mask TypeOptions cOutMin: Setpoint Weighting (Derivative)/OutMin | cOut/OutMin
      mask TypeOptions cOutMax: Setpoint Weighting (Derivative)/OutMax | cOut/OutMax
      mask TypeOptions cGainOutDataTypeStr: Setpoint Weighting (Derivative)/OutDataTypeStr
      mask TypeOptions cProdOutDataTypeStr: cOut/OutDataTypeStr
      mask TypeOptions KbOutMin: Kb/OutMin
      mask TypeOptions KbOutMax: Kb/OutMax
      mask TypeOptions KbOutDataTypeStr: Kb/OutDataTypeStr
      mask TypeOptions KtOutMin: Kt/OutMin
      mask TypeOptions KtOutMax: Kt/OutMax
      mask TypeOptions KtOutDataTypeStr: Kt/OutDataTypeStr
      mask TypeOptions IntegratorOutMin: Integrator/OutMin
      mask TypeOptions IntegratorOutMax: Integrator/OutMax
      mask TypeOptions IntegratorOutDataTypeStr: Integrator/OutDataTypeStr
      mask TypeOptions FilterOutMin: Filter/OutMin
      mask TypeOptions FilterOutMax: Filter/OutMax
      mask TypeOptions FilterOutDataTypeStr: Filter/OutDataTypeStr
      mask TypeOptions SumOutMin: Sum/OutMin
      mask TypeOptions SumOutMax: Sum/OutMax
      mask TypeOptions SumOutDataTypeStr: Sum/OutDataTypeStr
      mask TypeOptions Sum1OutMin: Sum1/OutMin
      mask TypeOptions Sum1OutMax: Sum1/OutMax
      mask TypeOptions Sum1OutDataTypeStr: Sum1/OutDataTypeStr
      mask TypeOptions Sum2OutMin: Sum2/OutMin
      mask TypeOptions Sum2OutMax: Sum2/OutMax
      mask TypeOptions Sum2OutDataTypeStr: Sum2/OutDataTypeStr
      mask TypeOptions Sum3OutMin: Sum3/OutMin
      mask TypeOptions Sum3OutMax: Sum3/OutMax
      mask TypeOptions Sum3OutDataTypeStr: Sum3/OutDataTypeStr
      mask TypeOptions SumI1OutMin: SumI1/OutMin
      mask TypeOptions SumI1OutMax: SumI1/OutMax
      mask TypeOptions SumI1OutDataTypeStr: SumI1/OutDataTypeStr
      mask TypeOptions SumI2OutMin: SumI2/OutMin
      mask TypeOptions SumI2OutMax: SumI2/OutMax
      mask TypeOptions SumI2OutDataTypeStr: SumI2/OutDataTypeStr
      mask TypeOptions SumI3OutMin: SumI3/OutMin
      mask TypeOptions SumI3OutMax: SumI3/OutMax
      mask TypeOptions SumI3OutDataTypeStr: SumI3/OutDataTypeStr
      mask TypeOptions SumDOutMin: SumD/OutMin
      mask TypeOptions SumDOutMax: SumD/OutMax
      mask TypeOptions SumDOutDataTypeStr: SumD/OutDataTypeStr
      mask TypeOptions SumAccumDataTypeStr: Sum/AccumDataTypeStr
      mask TypeOptions Sum1AccumDataTypeStr: Sum1/AccumDataTypeStr
      mask TypeOptions Sum2AccumDataTypeStr: Sum2/AccumDataTypeStr
      mask TypeOptions Sum3AccumDataTypeStr: Sum3/AccumDataTypeStr
      mask TypeOptions SumI1AccumDataTypeStr: SumI1/AccumDataTypeStr
      mask TypeOptions SumI2AccumDataTypeStr: SumI2/AccumDataTypeStr
      mask TypeOptions SumI3AccumDataTypeStr: SumI3/AccumDataTypeStr
      mask TypeOptions SumDAccumDataTypeStr: SumD/AccumDataTypeStr
      mask TypeOptions SaturationOutMin: Saturate/OutMin
      mask TypeOptions SaturationOutMax: Saturate/OutMax
      mask TypeOptions SaturationOutDataTypeStr: Saturate/OutDataTypeStr
      mask TypeOptions IntegratorContinuousStateAttributes: Integrator/ContinuousStateAttributes
      mask TypeOptions IntegratorStateIdentifier: Integrator/StateIdentifier
      mask TypeOptions IntegratorRTWStateStorageClass: Simulink:masks:Auto | Simulink:masks:ExportedGlobal | Simulink:masks:ImportedExtern | Simulink:masks:ImportedExternPointer
      mask TypeOptions FilterContinuousStateAttributes: Filter/ContinuousStateAttributes
      mask TypeOptions FilterStateIdentifier: Filter/StateIdentifier
      mask TypeOptions FilterRTWStateStorageClass: Simulink:masks:Auto | Simulink:masks:ExportedGlobal | Simulink:masks:ImportedExtern | Simulink:masks:ImportedExternPointer
      mask TypeOptions DifferentiatorICPrevScaledInput: Differentiator/UD/InitialCondition
      mask Display:
      | image(imread(fullfile(matlabroot,'toolbox','simulink','blocks','@pidpack','@PIDMasks','images','blank.png'),'png'),[0 0 1 1]);
      | disp('PID(s)')
      | port_label('input', 1, 'Ref');
      | port_label('input', 2, '');
      | port_label('output', 1, '');
  State-Space : StateSpace  X0=0
  Transfer Fcn : TransferFcn  Denominator=[1 1]
  Transport Delay : TransportDelay
  Variable Time Delay : VariableTransportDelay  MaximumDelay=10
  Variable Transport Delay : VariableTransportDelay  VariableDelayType=Variable transport delay  MaximumDelay=10
  Zero-Pole : ZeroPole  Poles=[0 -1]

== system intertravamento/Demos ==
